simulink model "sfunctestsim_2018a"  (R2018a)
settings: Solver=ode4  StartTime=0.0  StopTime=10.0  FixedStep=.01  RelTol=1e-3
settings Model: Creator=tdarrah  LastModifiedBy=tdarrah
settings DataIOCC: ReturnWorkspaceOutputs=on
settings SFSimCC: SimUseLocalCustomCode=on
settings RTWCC: RTWUseLocalCustomCode=on

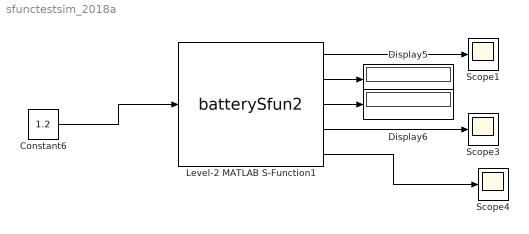
== system sfunctestsim_2018a ==
  Constant6 : Constant  Value=1.2
  Display5 : Display
  Display6 : Display
  Level-2 MATLAB S-Function1 : M-S-Function  FunctionName=batterySfun2  Parameters=battery, soc_ocv, .01
  Scope1 : Scope
  Scope3 : Scope
  Scope4 : Scope
  wires:
  Level-2 MATLAB S-Function1/1 -> Scope1/1
  Level-2 MATLAB S-Function1/4 -> Scope3/1
  Level-2 MATLAB S-Function1/5 -> Scope4/1
  Level-2 MATLAB S-Function1/2 -> Display5/1
  Level-2 MATLAB S-Function1/3 -> Display6/1
  Constant6/1 -> Level-2 MATLAB S-Function1/1
